simulink model "longitudinal_feedback"  (R2020a)
settings: Solver=VariableStepAuto  StartTime=0.0  StopTime=10  RelTol=1e-3
undefined symbols (not defined in the file): A, B, C, D, q_eta
settings Model: Creator=Lum  LastModifiedBy=Lum

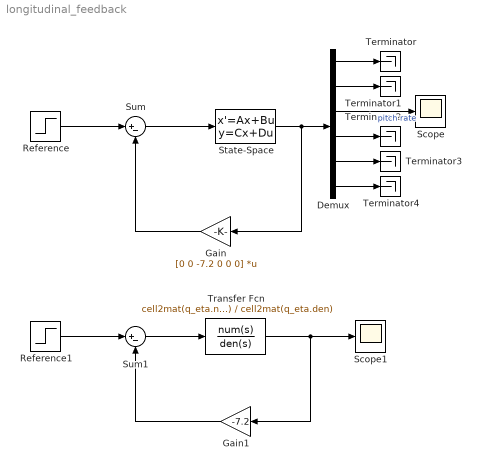
== system longitudinal_feedback ==
  Demux : Demux  Outputs=6
  Gain : Gain  Gain=[0 0 -7.2 0 0 0]  Multiplication=Matrix(K*u)
  Gain1 : Gain  Gain=-7.2
  Reference : Step  Time=0  After=deg2rad(1)  SampleTime=0
  Reference1 : Step  Time=0  After=deg2rad(1)  SampleTime=0
  Scope : Scope
  Scope1 : Scope
  State-Space : StateSpace  A=A  B=B  C=C  D=D  InitialCondition=0
  Sum : Sum  Inputs=|+-
  Sum1 : Sum  Inputs=|+-
  Terminator{,1..4} (5 alike) : Terminator
  Transfer Fcn : TransferFcn  Numerator=cell2mat(q_eta.num)  Denominator=cell2mat(q_eta.den)
  wires:
  State-Space/1 -> Gain/1, Demux/1
  Demux/3 -> Scope/1  "pitch rate"
  Demux/1 -> Terminator/1
  Demux/2 -> Terminator1/1
  Demux/4 -> Terminator2/1
  Demux/5 -> Terminator3/1
  Demux/6 -> Terminator4/1
  Reference/1 -> Sum/1
  Sum/1 -> State-Space/1
  Gain/1 -> Sum/2
  Transfer Fcn/1 -> Gain1/1, Scope1/1
  Reference1/1 -> Sum1/1
  Sum1/1 -> Transfer Fcn/1
  Gain1/1 -> Sum1/2
